simulink model "underactuatedBalancing"  (R2024a)
settings: Solver=ode45  StartTime=0.0  StopTime=tspan  RelTol=1e-8  AbsTol=1e-8
values from neighbouring files (symbols this model uses):
  C_f = 0.000    (= 0)    [pointMassTest.m]
  delta_d = [0.02 0.06 0]'    [Silva_SimulinkScript.m]    (also in pointMassTest.m = [0 0 0]')
  EA_0 = deg2rad([0 0 0]')    [Choi_SimulinkScript.m]    (also in SADS_UKF_Script.m = deg2rad([10 10 0]'); pointMassTest.m = [0 0 0]')
  g_N = [0 0 -9.81]    [Choi_SimulinkScript.m]    (also in SADS_UKF_Script.m; pointMassTest.m = [0 0 -9.81]')
  J_0 = [1.815  -0.014 0.004 ... (first row only)    [Choi_SimulinkScript.m]    (also in Silva_SimulinkScript.m = [0.265 -0.014 -0.035; -0.014 0.246 -0.018; -0.035 -0.018 0.4; pointMassTest.m = diag([0.0226, 0.0257 0.0266]))
  J_plat = J_0 - sum    [pointMassTest.m]
  k_p = 200    [Choi_SimulinkScript.m]    (also in pointMassTest.m = 0.01)
  m_i = 0.6    [pointMassTest.m]
  m_s = 33.629    [Choi_SimulinkScript.m]    (also in SADS_UKF_Script.m; pointMassTest.m = 4.2)
  q_0 = [0.99 -0.005 -0.063 -0.105]'    [Choi_SimulinkScript.m]    (also in SADS_UKF_Script.m = eul2quat(EA_0',"XYZ")'; Silva_SimulinkScript.m = [1 0 0 0]'; pointMassTest.m = [0 0 0 1]')
  r_b_0 = [-1 -3 -5]'*10^-3    [Silva_SimulinkScript.m]    (also in pointMassTest.m = [1 -0.9 -1.4]'.*1e-4)
  rho = [0 0 0 ... (first row only)    [pointMassTest.m]
  w_0 = [0 0 0.02]'    [pointMassTest.m]
undefined symbols (not defined in the file or in its folder): r_hat0
libraries: sharedtransform x2
settings Model: Creator=cocmc  LastModifiedBy=camer

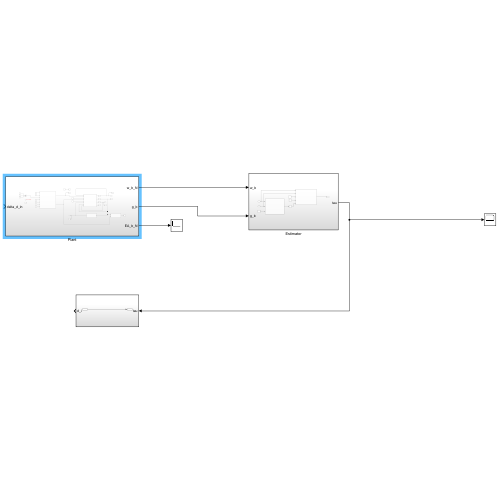
[thumbnail: Simulink's stored preview of the top-level diagram]
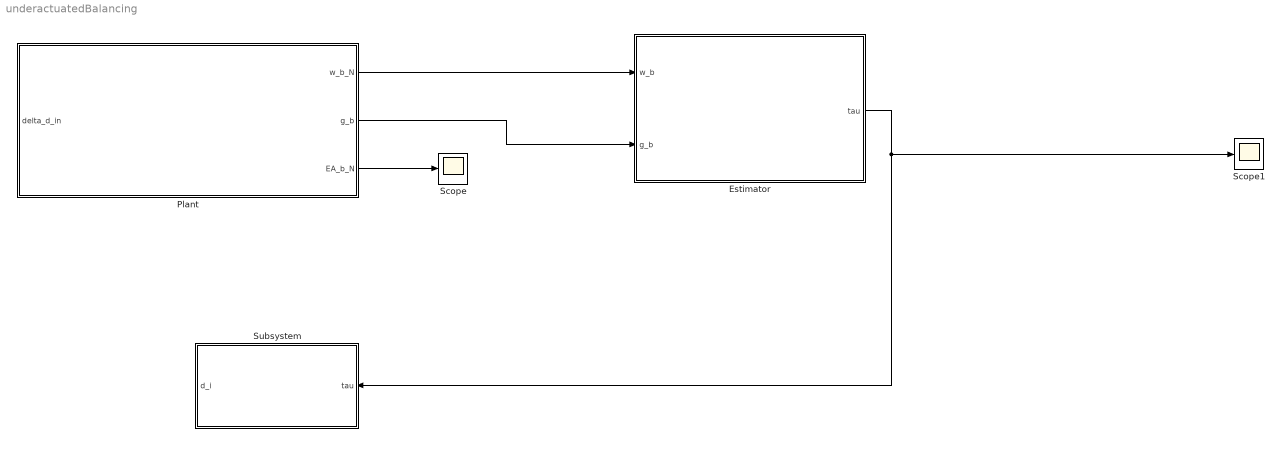
== system underactuatedBalancing ==
  Estimator : Subsystem
  Plant : Subsystem
  Scope : Scope
  Scope1 : Scope
  Subsystem : Subsystem
  wires:
  Plant/1(w_b_N) -> Estimator/1(w_b)
  Plant/2(g_b) -> Estimator/2(g_b)
  Estimator/1(tau) -> Scope1/1, Subsystem/1(tau)
  Plant/3(EA_b_N) -> Scope/1

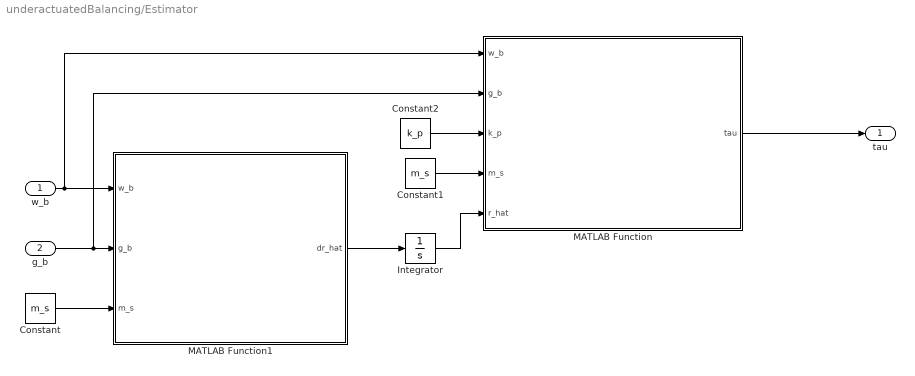
== system underactuatedBalancing/Estimator ==
  w_b : Inport
  g_b : Inport  Port=2
  Constant : Constant  Value=m_s
  Constant1 : Constant  Value=m_s
  Constant2 : Constant  Value=k_p
  Integrator : Integrator  InitialCondition=r_hat0
  MATLAB Function : MATLAB Function  TreatAsAtomicUnit=on
  MATLAB Function1 : MATLAB Function  TreatAsAtomicUnit=on
  tau : Outport
  wires:
  MATLAB Function/1(tau) -> tau/1
  w_b/1 -> MATLAB Function1/1(w_b), MATLAB Function/1(w_b)
  g_b/1 -> MATLAB Function/2(g_b), MATLAB Function1/2(g_b)
  Constant/1 -> MATLAB Function1/3(m_s)
  MATLAB Function1/1(dr_hat) -> Integrator/1
  Integrator/1 -> MATLAB Function/5(r_hat)
  Constant1/1 -> MATLAB Function/4(m_s)
  Constant2/1 -> MATLAB Function/3(k_p)

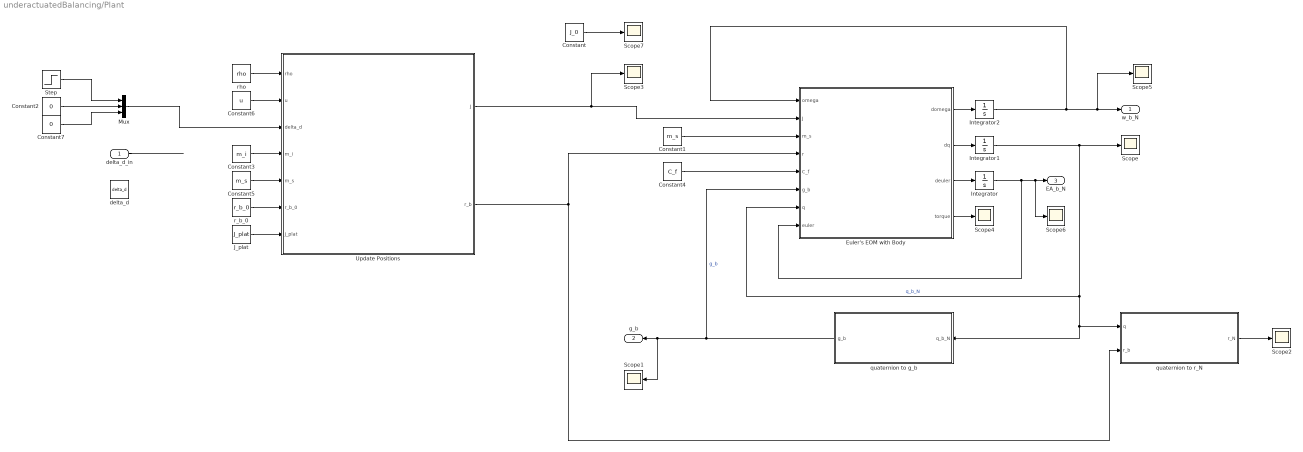
== system underactuatedBalancing/Plant ==
  delta_d_in : Inport
  Constant : Constant  Value=J_0
  Constant1 : Constant  Value=m_s
  Constant2 : Constant  Value=0
  Constant3 : Constant  Value=m_i
  Constant4 : Constant  Value=C_f
  Constant5 : Constant  Value=m_s
  Constant6 : Constant  Value=u
  Constant7 : Constant  Value=0
  Euler's EOM with Body : MATLAB Function  TreatAsAtomicUnit=on
  Integrator : Integrator  InitialCondition=EA_0
  Integrator1 : Integrator  InitialCondition=q_0
  Integrator2 : Integrator  InitialCondition=w_0
  J_plat : Constant  Value=J_plat
  Mux : Mux  Inputs=3
  Scope{,1..7} (8 alike) : Scope
  Step : Step  Time=10  After=0.010  SampleTime=0
  Update Positions : MATLAB Function  TreatAsAtomicUnit=on
  delta_d : Constant  Value=delta_d
  quaternion to g_b : Subsystem
  quaternion to r_N : Subsystem
  r_b_0 : Constant  Value=r_b_0
  rho : Constant  Value=rho
  w_b_N : Outport
  g_b : Outport  Port=2
  EA_b_N : Outport  Port=3
  wires:
  Constant1/1 -> Euler's EOM with Body/3(m_s)
  Euler's EOM with Body/1(domega) -> Integrator2/1
  Integrator2/1 -> Scope5/1, w_b_N/1, Euler's EOM with Body/1(omega)
  Euler's EOM with Body/3(deuler) -> Integrator/1
  Integrator/1 -> Euler's EOM with Body/8(euler), Scope6/1, EA_b_N/1
  Euler's EOM with Body/2(dq) -> Integrator1/1
  Integrator1/1 -> quaternion to g_b/1(q_b_N), quaternion to r_N/1(q), Euler's EOM with Body/7(q), Scope/1  "q_b_N"
  quaternion to g_b/1(g_b) -> Scope1/1, g_b/1, Euler's EOM with Body/6(g_b)  "g_b"
  Constant4/1 -> Euler's EOM with Body/5(C_f)
  quaternion to r_N/1(r_N) -> Scope2/1
  Euler's EOM with Body/4(torque) -> Scope4/1
  delta_d_in/1 -> ?
  Constant6/1 -> Update Positions/2(u)
  rho/1 -> Update Positions/1(rho)
  Constant3/1 -> Update Positions/4(m_i)
  Constant5/1 -> Update Positions/5(m_s)
  r_b_0/1 -> Update Positions/6(r_b_0)
  Update Positions/2(r_b) -> quaternion to r_N/2(r_b), Euler's EOM with Body/4(r)
  J_plat/1 -> Update Positions/7(J_plat)
  Update Positions/1(J) -> Scope3/1, Euler's EOM with Body/2(J)
  Constant/1 -> Scope7/1
  Constant2/1 -> Mux/2
  Constant7/1 -> Mux/3
  Step/1 -> Mux/1
  Mux/1 -> Update Positions/3(delta_d)

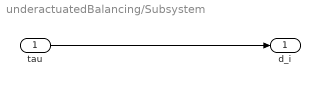
== system underactuatedBalancing/Subsystem ==
  tau : Inport
  d_i : Outport
  wires:
  tau/1 -> d_i/1

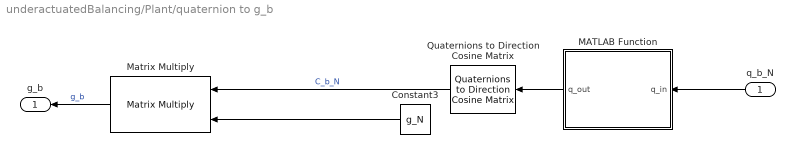
== system underactuatedBalancing/Plant/quaternion to g_b ==
  q_b_N : Inport
  Constant3 : Constant  Value=g_N
  MATLAB Function : MATLAB Function  TreatAsAtomicUnit=on
  Matrix Multiply : Product  Multiplication=Matrix(*)
  Quaternions to Direction Cosine Matrix : sharedtransform/Quaternions to  Direction Cosine Matrix  aMode=aMode
      settings: LibrarySourceBlock=|
      | aerolibtransform2/Quaternions to
      | Direction Cosine Matrix
  g_b : Outport
  wires:
  Constant3/1 -> Matrix Multiply/2
  MATLAB Function/1(q_out) -> Quaternions to Direction Cosine Matrix/1
  Quaternions to Direction Cosine Matrix/1 -> Matrix Multiply/1  "C_b_N"
  q_b_N/1 -> MATLAB Function/1(q_in)
  Matrix Multiply/1 -> g_b/1  "g_b"

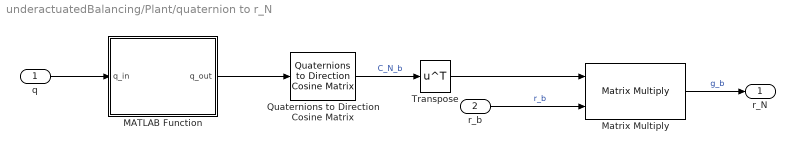
== system underactuatedBalancing/Plant/quaternion to r_N ==
  q : Inport
  r_b : Inport  Port=2
  MATLAB Function : MATLAB Function  TreatAsAtomicUnit=on
  Matrix Multiply : Product  Multiplication=Matrix(*)
  Quaternions to Direction Cosine Matrix : sharedtransform/Quaternions to  Direction Cosine Matrix  aMode=aMode
      settings: LibrarySourceBlock=|
      | aerolibtransform2/Quaternions to
      | Direction Cosine Matrix
  Transpose : Math  Operator=transpose
  r_N : Outport
  wires:
  r_b/1 -> Matrix Multiply/2  "r_b"
  MATLAB Function/1(q_out) -> Quaternions to Direction Cosine Matrix/1
  Quaternions to Direction Cosine Matrix/1 -> Transpose/1  "C_N_b"
  q/1 -> MATLAB Function/1(q_in)
  Matrix Multiply/1 -> r_N/1  "g_b"
  Transpose/1 -> Matrix Multiply/1

== matlab function underactuatedBalancing/Estimator/MATLAB Function1 ==
  data: w_b input; dr_hat output; g_b input; m_s input
function dr_hat = fcn(w_b,g_b,m_s)

g_cross =  [0      -g_b(3)  g_b(2);
            g_b(3)  0      -g_b(1);
           -g_b(2)  g_b(1)  0 ];

kappa = -m_s*g_cross;

dr_hat = -kappa'*w_b;

== matlab function underactuatedBalancing/Estimator/MATLAB Function ==
  data: w_b input; tau output; g_b input; k_p input; m_s input; r_hat input
function tau = fcn(w_b,g_b,k_p,m_s,r_hat)

P = eye(3) - (g_b*g_b') / (norm(g_b)^2);

w_p = P*w_b;

tau = m_s*(cross(g_b,r_hat)) - k_p*w_p;

== matlab function underactuatedBalancing/Plant/Euler's EOM with Body ==
  data: omega input; J input; m_s input; r input; C_f input; g_b input; q input; domega output; euler input; dq output; deuler output; torque output
function [domega,dq,deuler,torque] = fcn(omega,J,m_s,r,C_f,g_b,q,euler)

% C_b_N = [1 - 2*(q(2)^2 + q(3)^2), 2*(q(1)*q(2) - q(4)*q(3)), 2*(q(1)*q(3) + q(4)*q(2));
%    2*(q(1)*q(2) + (q(4)*q(3))), 1 - 2*(q(1)^2 + q(3)^2), 2*(q(2)*q(3) - q(4)*q(1));
%     2*(q(1)*q(3) - q(4)*q(2)),  2*(q(1)*q(3) + q(4)*q(1)),  1 - 2*(q(1)^2 + q(2)^2)];

% g_b = C_b_N*[0 0 -9.81]';

g_b_cross = [0        -g_b(3) g_b(2);
            g_b(3)  0         -g_b(1);
           -g_b(2)  g_b(1) 0 ];

torque = cross(r,m_s*g_b) - C_f.*omega;

omega_cross = [0        -omega(3) omega(2);
            omega(3)  0         -omega(1);
           -omega(2)  omega(1) 0 ];



% equations of motion
domega = J\(torque - omega_cross*(J*omega));

% domega = torque./J(1,1);
% domega = [0 0 0]';

% propogating kinematics...
Phi = euler(1);
Theta = euler(2);
Psi = euler(3);

matrix = (1/cos(Theta)).*[cos(Theta) sin(Phi)*sin(Theta)  cos(Phi)*sin(Theta);
                              0          cos(Phi)*cos(Theta) -sin(Phi)*cos(Theta);
                              0          sin(Phi)             cos(Phi)];

product = matrix * omega;

dPhi = product(1);
dTheta = product(2);
dPsi = product(3);

deuler = [dPhi dTheta dPsi]';

epsilon = [q(1) q(2) q(3)];
eta = q(4);

crossvec = [0          -epsilon(3) epsilon(2);
            epsilon(3)  0         -epsilon(1);
           -epsilon(2)  epsilon(1) 0 ];

dEta = (-1/2)*(epsilon*omega);
dEpsilon = (1/2)*((eta*eye(3)) + crossvec)*omega;

dEpsilon1 = dEpsilon(1);
dEpsilon2 = dEpsilon(2);
dEpsilon3 = dEpsilon(3);

% dq = [dEpsilon1 dEpsilon2 dEpsilon3 dEta]';
dq = 1/2*[0 omega(3) -omega(2) omega(1);     -omega(3) 0 omega(1) omega(2);    omega(2) -omega(1) 0 omega(3);    -omega(1) -omega(2) -omega(3)    0]*q;

== matlab function underactuatedBalancing/Plant/quaternion to r_N/MATLAB Function ==
  data: q_in input; q_out output
function q_out = moveEtaFirst(q_in)

q_out = [q_in(4) q_in(1) q_in(2) q_in(3)];

== matlab function underactuatedBalancing/Plant/quaternion to g_b/MATLAB Function ==
  data: q_in input; q_out output
function q_out = moveEtaFirst(q_in)

q_out = [q_in(4) q_in(1) q_in(2) q_in(3)];

== matlab function underactuatedBalancing/Plant/Update Positions ==
  data: J output; rho input; r_b output; u input; delta_d input; m_i input; m_s input; r_b_0 input; J_plat input
function [J,r_b] = fcn(rho,u,delta_d,m_i,m_s,r_b_0,J_plat)

sum = zeros(size(u,2), 1);
for i = 1:size(u,2)
    sum = sum + m_i*delta_d(i)*u(:,i);
end
del_r_b = (1/m_s)*sum;
r_b = r_b_0 + del_r_b;

sum = zeros(size(rho,2),size(rho,2));
for i = 1:size(rho,2)
    R_i = rho(:,i) + delta_d(i)*u(:,i);
    R_i_cross = [0 -R_i(3) R_i(2);
                 R_i(3) 0 -R_i(1);
                -R_i(2) R_i(1) 0];
    sum = sum - (m_i*R_i_cross*R_i_cross);
end

J = J_plat + sum;
